simulink model "vehicle_SSC"  (R2022a)
settings: Solver=VariableStepAuto  StartTime=0.0  StopTime=10.0  RelTol=1e-3
PreLoadFcn:
  | vehicleObject = vehicle.ParallelSUV;
libraries: fl_lib x21, nesl_utility x9, sdl_lib x6
settings Model: Creator=grouleau  LastModifiedBy=grouleau

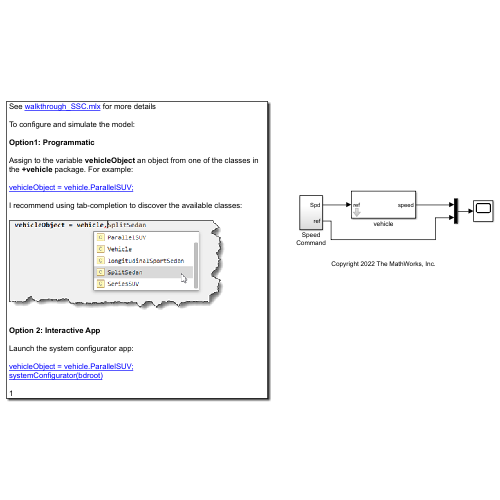
[thumbnail: Simulink's stored preview of the top-level diagram]
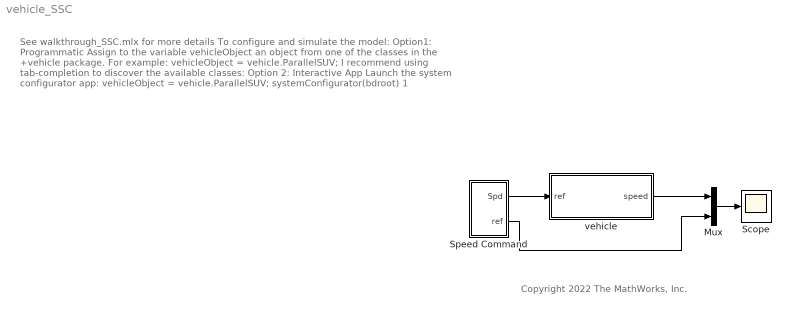
== system vehicle_SSC ==
  note: See walkthrough_SSC.mlx for more details
      |
      | To configure and simulate the model:
      |
      | Option1: Programmatic
      |
      | Assign to the variable vehicleObject an object from one of the classes in the +vehicle package. For example:
      |
      | vehicleObject = vehicle.ParallelSUV;
      |
      | I recommend using tab-completion to discover the available classes:
      |
      | Option 2: Interactive App
      |
      | Launch the system configurator app:
      |
      | vehicleObject = vehicle.ParallelSUV;
      | systemConfigurator(bdroot)
      |
      | 1
  note: Copyright 2022 The MathWorks, Inc.
  Mux : Mux  Inputs=2
  Scope : Scope
  Speed Command : Subsystem
  vehicle : Subsystem  mask(slPart){obj=vehicleObject}
      mask prompts: obj "slPart Object:"
      mask help: This subsystem implements a simplified vehicle with multiple hybrid drivetrain and parameterizations. To configure the vehicle, assign an object instantiated from one of the class in the "+vehicle" folder.
      mask init:
      | obj.maskInit(gcb);
      mask DialogControl Control2 Prompt: See walkthrough_SSC.mlx for more examples
      mask DialogControl Control2 Callback: open('walkthrough_SSC.mlx')
      mask DialogControl Container3 Prompt: Example
      mask DialogControl Control3 Prompt: vehicleObject = vehicle.ParallelSUV;
      mask DialogControl Control3 Callback: vehicleObject = vehicle.ParallelSUV;
  wires:
  Speed Command/1(Spd) -> vehicle/1(ref)
  Mux/1 -> Scope/1
  vehicle/1(speed) -> Mux/1
  Speed Command/2(ref) -> Mux/2

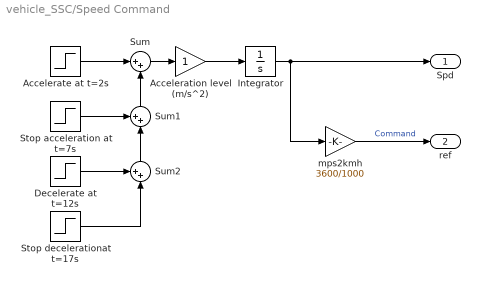
== system vehicle_SSC/Speed Command ==
  Accelerate at t=2s : Step  Time=2  SampleTime=0
  Acceleration level (m/s^2) : Gain
  Decelerate at t=12s : Step  Time=12  After=-1  SampleTime=0
  Integrator : Integrator  InitialCondition=15
  Stop acceleration at t=7s : Step  Time=7  After=-1  SampleTime=0
  Stop decelerationat t=17s : Step  Time=17  SampleTime=0
  Sum : Sum  Inputs=|++
  Sum1 : Sum  Inputs=++|
  Sum2 : Sum  Inputs=++|
  mps2kmh : Gain  Gain=3600/1000
  Spd : Outport  VectorParamsAs1DForOutWhenUnconnected=off
  ref : Outport  Port=2  VectorParamsAs1DForOutWhenUnconnected=off
  wires:
  Integrator/1 -> mps2kmh/1, Spd/1
  mps2kmh/1 -> ref/1  "Command"
  Stop decelerationat t=17s/1 -> Sum2/2
  Decelerate at t=12s/1 -> Sum2/1
  Acceleration level (m/s^2)/1 -> Integrator/1
  Sum2/1 -> Sum1/2
  Sum1/1 -> Sum/2
  Stop acceleration at t=7s/1 -> Sum1/1
  Sum/1 -> Acceleration level (m/s^2)/1
  Accelerate at t=2s/1 -> Sum/1

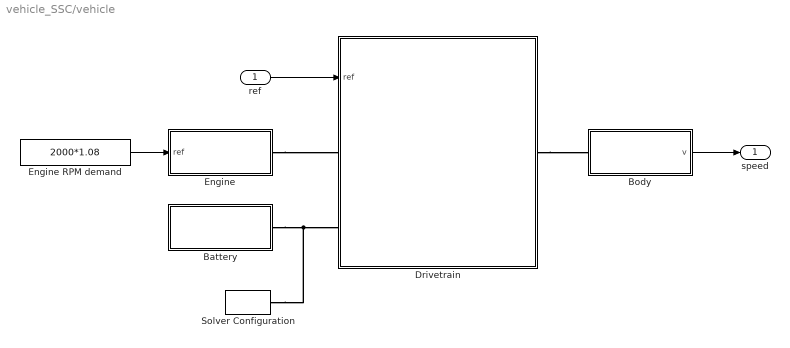
== system vehicle_SSC/vehicle ==
  ref : Inport
  Battery : Subsystem  mask(slPart){obj=obj.Battery}
      mask prompts: obj "slPart Object:"
      mask help: Container block for all slPart blocks
      mask init:
      | obj.maskInit(gcb);
  Body : Subsystem  mask(slPart){obj=obj.Body}
      mask prompts: obj "slPart Object:"
      mask help: Container block for all slPart blocks
      mask init:
      | obj.maskInit(gcb);
  Drivetrain : Subsystem  Variant=on  VariantControlMode=label  LabelModeActiveChoice=drivetrain.Parallel  mask(slPart){obj=obj.Drivetrain}
      mask prompts: obj "slPart Object:"
      mask help: Container block for all slPart blocks
      mask init:
      | obj.maskInit(gcb);
  Engine : Subsystem  mask(slPart){obj=obj.Engine}
      mask prompts: obj "slPart Object:"
      mask help: Container block for all slPart blocks
      mask init:
      | obj.maskInit(gcb);
  Engine RPM demand : Constant  Value=2000*1.08
  Solver Configuration : nesl_utility/Solver Configuration  PhysicalDomain=network_engine_domain  SubClassName=solver  LeftPortType=input  RightPortType=generic  Tones=[]  Harmonics=[]  SimulateNoise=off  Profile=off  UseLocalSampling=off  EnableSwitchedLinearOptims=on  FrequencyDomain=off  UseCCode=off  RelTol=0.001  AbsTol=1e-06  MinStep=1e-09  ToWorkspace=off  RevertToSquareIcSolve=off  NumHomotopyIterations=100  PhasorMode=off  PhasorModeNumHarmonics=1  IndexReductionMethod=DerivativeReplacement  DoDC=off  ResidualTolerance=1e-9  UseLocalSolver=off  LocalSolverChoice=NE_PARTITIONING_ADVANCER  LocalSolverSampleTime=0.005  DoFixedCost=off  MaxNonlinIter=5  MaxModeIter=2  ComputeImpulses=off  ImpulseIterations=2  LinearAlgebra=auto  LinearAlgebraNumThread=0  EquationFormulation=NE_TIME_EF  DelaysMemoryBudget=1024  AutomaticFiltering=on  FilteringTimeConstant=0.001  PartitionStorageMethod=EXHAUSTIVE  PartitionMemoryBudget=1024  PartitionMethod=ROBUST
      settings: SourceProductBaseCode=PW,SS
  speed : Outport
  wires:
  Body/1(v) -> speed/1
  ref/1 -> Drivetrain/1(ref)
  Engine RPM demand/1 -> Engine/1(ref)
  connections:
  Engine/RConn1 -- Drivetrain/LConn1
  Battery/RConn1 -- Solver Configuration/RConn1 -- Drivetrain/LConn2
  Drivetrain/RConn1 -- Body/LConn1

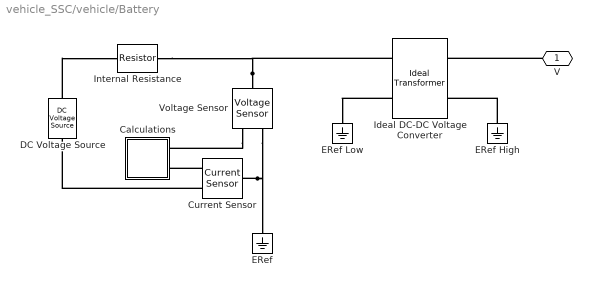
== system vehicle_SSC/vehicle/Battery ==
  Calculations : Subsystem
  Current Sensor : fl_lib/Electrical/Electrical Sensors/Current Sensor
  DC Voltage Source : fl_lib/Electrical/Electrical Sources/DC Voltage Source  v0=obj.BatteryVoltage V
  ERef : fl_lib/Electrical/Electrical Elements/Electrical Reference
  ERef High : fl_lib/Electrical/Electrical Elements/Electrical Reference
  ERef Low : fl_lib/Electrical/Electrical Elements/Electrical Reference
  Ideal DC-DC Voltage Converter : fl_lib/Electrical/Electrical Elements/Ideal Transformer  n=obj.OutputVoltage/obj.BatteryVoltage  i1_specify=off  i1_priority=None  i1=0 A  i1_nominal_specify=off  i1_nominal_unit=A  i1_nominal_value=1  v1_specify=off  v1_priority=None  v1=0 V  v1_nominal_specify=off  v1_nominal_unit=V  v1_nominal_value=1  i2_specify=off  i2_priority=None  i2=0 A  i2_nominal_specify=off  i2_nominal_unit=A  i2_nominal_value=1  v2_specify=off  v2_priority=None  v2=0 V  v2_nominal_specify=off  v2_nominal_unit=V  v2_nominal_value=1
      settings: SourceProductBaseCode=SS
  Internal Resistance : fl_lib/Electrical/Electrical Elements/Resistor  R=0.05 Ohm  i_specify=off  i_priority=High  i=0 A  i_nominal_specify=off  i_nominal_unit=A  i_nominal_value=1  v_specify=off  v_priority=High  v=0 V  v_nominal_specify=off  v_nominal_unit=V  v_nominal_value=1
  Voltage Sensor : fl_lib/Electrical/Electrical Sensors/Voltage Sensor
  V : PMIOPort  Side=Right
  connections:
  Current Sensor/LConn1 -- ERef/LConn1 -- Voltage Sensor/RConn2
  Voltage Sensor/LConn1 -- Internal Resistance/RConn1 -- Ideal DC-DC Voltage Converter/LConn1
  Current Sensor/RConn2 -- DC Voltage Source/RConn1
  Ideal DC-DC Voltage Converter/LConn2 -- ERef Low/LConn1
  Voltage Sensor/RConn1 -- Calculations/LConn1
  DC Voltage Source/LConn1 -- Internal Resistance/LConn1
  ERef High/LConn1 -- Ideal DC-DC Voltage Converter/RConn2
  Current Sensor/RConn1 -- Calculations/LConn2
  V/RConn1 -- Ideal DC-DC Voltage Converter/RConn1

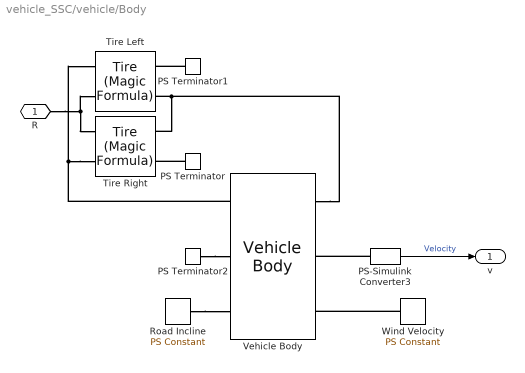
== system vehicle_SSC/vehicle/Body ==
  PS Terminator : fl_lib/Physical Signals/Sinks/PS Terminator
      settings: SourceProductBaseCode=PW,SS,VE
  PS Terminator1 : fl_lib/Physical Signals/Sinks/PS Terminator
      settings: SourceProductBaseCode=PW,SS,VE
  PS Terminator2 : fl_lib/Physical Signals/Sinks/PS Terminator
      settings: SourceProductBaseCode=PW,SS,VE
  PS-Simulink Converter3 : nesl_utility/PS-Simulink Converter  PhysicalDomain=network_engine_domain  SubClassName=ps_output  LeftPortType=input  RightPortType=output  PseudoPeriodic=off  Frequencies=[]  VectorFormat=1-D array  Unit=km/hr  AffineConversion=off
      settings: SourceProductBaseCode=PW,SS
  Road Incline : fl_lib/Physical Signals/Sources/PS Constant  constant=0
  Tire Left : sdl_lib/Tires & Vehicles/Tire (Magic Formula)  parameterization=sdl.enum.magic_tire_model.peak  F_z1=3000 N  F_x1=3500 N  kappa1=10  B_m=10  C_m=1.9  D_m=1  E_m=0.97  fz0=4e+3 N  p_Cx=1.685  p_Dx=[ 1.21 -0.037 ]  p_Ex=[ 0.344 0.095 -0.02 0 ]  p_Kx=[ 21.51 -0.163 0.245 ]  p_Hx=[ -0.002 0.002 ]  p_Vx=[ 0 0 ]  r_e=obj.WheelRadius m  model_compliance=sdl.enum.compliance.off  stiffness=1e+6 N/m  damping=1000 N/(m/s)  model_inertia=sdl.enum.model_inertia.on  inertia=1e-2 kg*m^2  initial_velocity=obj.InitialVelocity/obj.WheelRadius rad/s  model_resistance=simscape.enum.onoff.off  resistance_model=sdl.enum.rollingResistanceParameterization.constant  coeff=0.015  p_tire=2.5e+5 Pa  alpha=-0.003  beta=0.97  coeff_a=0.008399999999999999  coeff_b=6.2e-4 s/m  coeff_c=1.6e-4 s^2/m^2  v_thr=0.001 m/s  v_tr_thr=0.1 m/s
  Tire Right : sdl_lib/Tires & Vehicles/Tire (Magic Formula)  parameterization=sdl.enum.magic_tire_model.peak  F_z1=3000 N  F_x1=3500 N  kappa1=10  B_m=10  C_m=1.9  D_m=1  E_m=0.97  fz0=4e+3 N  p_Cx=1.685  p_Dx=[ 1.21 -0.037 ]  p_Ex=[ 0.344 0.095 -0.02 0 ]  p_Kx=[ 21.51 -0.163 0.245 ]  p_Hx=[ -0.002 0.002 ]  p_Vx=[ 0 0 ]  r_e=obj.WheelRadius m  model_compliance=sdl.enum.compliance.off  stiffness=1e+6 N/m  damping=1000 N/(m/s)  model_inertia=sdl.enum.model_inertia.on  inertia=1e-2 kg*m^2  initial_velocity=obj.InitialVelocity/obj.WheelRadius rad/s  model_resistance=simscape.enum.onoff.off  resistance_model=sdl.enum.rollingResistanceParameterization.constant  coeff=0.015  p_tire=2.5e+5 Pa  alpha=-0.003  beta=0.97  coeff_a=0.008399999999999999  coeff_b=6.2e-4 s/m  coeff_c=1.6e-4 s^2/m^2  v_thr=0.001 m/s  v_tr_thr=0.1 m/s
  Vehicle Body : sdl_lib/Tires & Vehicles/Vehicle Body  mass=obj.Mass kg  n_w=2  x_f=1.4 m  x_r=1.6 m  y_c=0.5 m  mass_var=simscape.enum.onoff.off  g=9.81 m/s^2  liftoff_warning=simscape.enum.onoff.off  area=3 m^2  Cd=0.4  rho=1.18 kg/m^3  model_pitch=simscape.enum.onoff.off  inertia=4000 kg*m^2  suspension_model=sdl.enum.linearTLU.linear  k_f=1e4 N/m  b_f=1e4 N/(m/s)  k_r=1e4 N/m  b_r=1e4 N/(m/s)  k_f_TLU=[-2000, -1000, 0, 1000, 2000] N  x_f_TLU=[-.4, -.2, 0, .2, .4] m  b_f_TLU=[-200, -100, 0, 100, 200] N  v_f_TLU=[-4, -2, 0, 2, 4] m/s  k_r_TLU=[-2000, -1000, 0, 1000, 2000] N  x_r_TLU=[-.4, -.2, 0, .2, .4] m  b_r_TLU=[-200, -100, 0, 100, 200] N  v_r_TLU=[-4, -2, 0, 2, 4] m/s  interp_method=simscape.enum.interpolation.linear  extrap_method=simscape.enum.extrapolation.linear  model_hardstop=simscape.enum.onoff.off  upper_bound_f=.25 m  lower_bound_f=-.25 m  stop_k_f=1e6 N/m  stop_b_f=150 N/(m/s)  upper_bound_r=.25 m  lower_bound_r=-.25 m  stop_k_r=1e6 N/m  stop_b_r=150 N/(m/s)  initial_pitch=0 rad  initial_pitch_rate=0 rad/s  v_specify=on  v_priority=High  v=obj.InitialVelocity m/s  v_nominal_specify=off  v_nominal_unit=m/s  v_nominal_value=1
  Wind Velocity : fl_lib/Physical Signals/Sources/PS Constant  constant=0
  R : PMIOPort  Side=Left
  v : Outport  VectorParamsAs1DForOutWhenUnconnected=off
  wires:
  PS-Simulink Converter3/1 -> v/1  "Velocity"
  connections:
  Vehicle Body/LConn1 -- Tire Right/RConn2 -- Tire Left/RConn2
  R/RConn1 -- Tire Left/LConn2 -- Tire Right/LConn2
  Tire Right/LConn1 -- Tire Left/LConn1 -- Vehicle Body/RConn1
  Wind Velocity/RConn1 -- Vehicle Body/LConn3
  Road Incline/RConn1 -- Vehicle Body/RConn3
  PS-Simulink Converter3/LConn1 -- Vehicle Body/LConn2
  PS Terminator/LConn1 -- Tire Right/RConn1
  PS Terminator1/LConn1 -- Tire Left/RConn1
  PS Terminator2/LConn1 -- Vehicle Body/RConn2

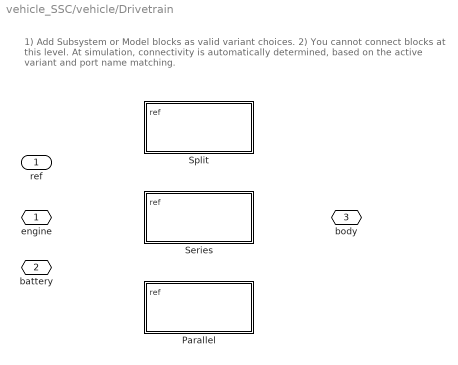
== system vehicle_SSC/vehicle/Drivetrain ==
  note: 1) Add Subsystem or Model blocks as valid variant choices.
      | 2) You cannot connect blocks at this level. At simulation, connectivity is automatically
      | determined, based on the active variant and port name matching.
  ref : Inport
  Parallel : Subsystem  VariantControl=drivetrain.Parallel
  Series : Subsystem  VariantControl=drivetrain.Series
  Split : Subsystem  VariantControl=drivetrain.Split
  engine : PMIOPort  Side=Left
  battery : PMIOPort  Port=2  Side=Left
  body : PMIOPort  Port=3  Side=Right

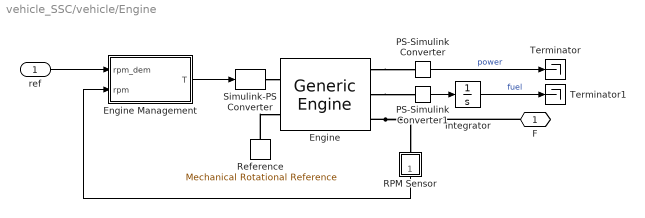
== system vehicle_SSC/vehicle/Engine ==
  ref : Inport
  Engine : sdl_lib/Engines & Motors/Generic Engine  model_parameterization=sdl.enum.engineParameterization.polynomial  engine_type=sdl.enum.engineType.SI  P_max=obj.MaximumPower kW  w_P_max=5500 rpm  w_max=7000 rpm  w_min=500 rpm  w_tab=[ 500 1000 2e+3 3e+3 4e+3 5e+3 6e+3 7e+3 ] rpm  trq_tab=[ 380 380 380 380 350 280 200 80 ] N*m  pwr_tab=[ 2e+4 4e+4 7.8e+4 1.2e+5 1.45e+5 1.48e+5 1.25e+5 6e+4 ] W  interp_method=simscape.enum.interpolation.linear  model_inertia=sdl.enum.model_inertia.on  inertia=0.2 kg*m^2  initial_velocity=obj.Initial_rpm rpm  model_time_constant=sdl.enum.lagOffOn.on  time_constant=0.2 s  T0=0.15  w_thr=20 rpm  fc_model=sdl.enum.fuel_consumption_model.BSFCSpeedBMEP  fc_per_rev=25 mg/rev  fc_w_tab=[ 1000 2e+3 3e+3 4e+3 5e+3 6e+3 ] rpm  fc_trq_tab=[ 0 80 160 200 240 320 360 400 ] N*m  fc_tab=[ 0.5 0.9 1.4 1.6 1.9 2.7 3.4 4.4; 1 1.7 2.7 3.1 3.6 5 6 7.4; 1.4 2.7 4 4.8 5.6 7.5 8.5 10.5; 2 3.6 5.8 6.7 8 10.4 11.7 13.3; 2.5 4.8 7.9 9.4 10.8 14 16.2 18.6; 3.1 6 10.3 11.9 13.8 18.4 22 26.5 ] g/s  bmep_tab=[ 0 250 500 625 750 1000 1.15e+3 1.25e+3 ] kPa  bsfc_tab=[ 410 380 300 280 270 290 320 380; 410 370 290 270 260 270 285 320; 415 380 290 275 265 270 270 300; 420 390 310 290 285 280 280 285; 430 410 340 320 310 300 310 320; 450 430 370 340 330 330 350 380 ] g/(hr*kW)  fc_interp_method=simscape.enum.interpolation.linear  idle_speed=simscape.enum.onoff.off  idle_speed_reference=1000 rpm  tau_controller=1 s  idle_w_thr=1 rpm  redline=simscape.enum.onoff.off  redline_speed=5000 rpm  tau_redline=1 s  redline_w_thr=1 rpm  displaced_volume=400 cm^3  rev_per_cycle=2
      settings: SourceProductBaseCode=LD  InternalSimscapePortConfiguration="{\"Bottom\":[],\"Left\":[{\"id\":\"T\",\"label\":\"T\",\"type\":\"input\"},{\"id\":\"B\",\"label\":\"B\",\"type\":\"foundation.mechanical.rotational.rotational\"}],\"Right\":[{\"id\":\"P\",\"label\":\"P\",\"type\":\"output\"},{\"id\":\"FC\",\"label\":\"FC\",\"type\":\"output\"},{\"id\":\"F\",\"label\":\"F\",\"type\":\"foundation.mechanical.rotational.rotational\"}],\"Top\":[]}"
  Engine Management : Subsystem
  Integrator : Integrator
  PS-Simulink Converter : nesl_utility/PS-Simulink Converter  PhysicalDomain=network_engine_domain  SubClassName=ps_output  LeftPortType=input  RightPortType=output  PseudoPeriodic=off  Frequencies=[]  VectorFormat=1-D array  Unit=inherit  AffineConversion=off
      settings: SourceProductBaseCode=PW,SS
  PS-Simulink Converter1 : nesl_utility/PS-Simulink Converter  PhysicalDomain=network_engine_domain  SubClassName=ps_output  LeftPortType=input  RightPortType=output  PseudoPeriodic=off  Frequencies=[]  VectorFormat=1-D array  Unit=inherit  AffineConversion=off
      settings: SourceProductBaseCode=PW,SS
  RPM Sensor : Subsystem
      mask Display: disp('S');
  Reference : fl_lib/Mechanical/Rotational Elements/Mechanical Rotational Reference
  Simulink-PS Converter : nesl_utility/Simulink-PS Converter  PhysicalDomain=network_engine_domain  SubClassName=ps_input  LeftPortType=input  RightPortType=output  PseudoPeriodic=off  Frequencies=[]  NoiseDistribution=none  NoiseParameters=[]  Unit=1  AffineConversion=off  FilteringAndDerivatives=zero  SimscapeFilterOrder=1  InputFilterTimeConstant=.001  UdotUserProvided=0
      settings: SourceProductBaseCode=PW,SS
  Terminator : Terminator
  Terminator1 : Terminator
  F : PMIOPort  Side=Right
  wires:
  Integrator/1 -> Terminator1/1  "fuel"
  RPM Sensor/1(rpm) -> Engine Management/2(rpm)
  Engine Management/1(T) -> Simulink-PS Converter/1
  PS-Simulink Converter/1 -> Terminator/1  "power"
  PS-Simulink Converter1/1 -> Integrator/1
  ref/1 -> Engine Management/1(rpm_dem)
  connections:
  Simulink-PS Converter/RConn1 -- Engine/LConn1
  Engine/RConn1 -- PS-Simulink Converter/LConn1
  Engine/RConn2 -- PS-Simulink Converter1/LConn1
  Reference/LConn1 -- Engine/LConn2
  Engine/RConn3 -- RPM Sensor/LConn1 -- F/RConn1

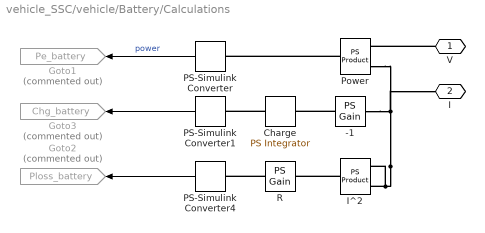
== system vehicle_SSC/vehicle/Battery/Calculations ==
  -1 : fl_lib/Physical Signals/Functions/PS Gain  gain=-1
  Charge : fl_lib/Physical Signals/Linear Operators/PS Integrator  reset_method=foundation.enum.IntegratorResetSpec.None  initial_condition_spec=foundation.enum.IntegratorICSpec.Internal  x0=150 A*hr
      settings: SourceProductBaseCode=SS
  Goto1 : Goto  Commented=on  GotoTag=Pe_battery  TagVisibility=global
  Goto2 : Goto  Commented=on  GotoTag=Ploss_battery  TagVisibility=global
  Goto3 : Goto  Commented=on  GotoTag=Chg_battery  TagVisibility=global
  I^2 : fl_lib/Physical Signals/Functions/PS Product
  PS-Simulink Converter : nesl_utility/PS-Simulink Converter  PhysicalDomain=network_engine_domain  SubClassName=ps_output  LeftPortType=input  RightPortType=output  PseudoPeriodic=off  Frequencies=[]  VectorFormat=1-D array  Unit=kW  AffineConversion=off
      settings: SourceProductBaseCode=PW,SS
  PS-Simulink Converter1 : nesl_utility/PS-Simulink Converter  PhysicalDomain=network_engine_domain  SubClassName=ps_output  LeftPortType=input  RightPortType=output  PseudoPeriodic=off  Frequencies=[]  VectorFormat=1-D array  Unit=A*hr  AffineConversion=off
      settings: SourceProductBaseCode=PW,SS
  PS-Simulink Converter4 : nesl_utility/PS-Simulink Converter  PhysicalDomain=network_engine_domain  SubClassName=ps_output  LeftPortType=input  RightPortType=output  PseudoPeriodic=off  Frequencies=[]  VectorFormat=1-D array  Unit=kW  AffineConversion=off
      settings: SourceProductBaseCode=PW,SS
  Power : fl_lib/Physical Signals/Functions/PS Product
  R : fl_lib/Physical Signals/Functions/PS Gain  gain=0.05 V/A
  V : PMIOPort  Side=Left
  I : PMIOPort  Port=2  Side=Left
  wires:
  PS-Simulink Converter4/1 -> Goto2/1
  PS-Simulink Converter1/1 -> Goto3/1
  PS-Simulink Converter/1 -> Goto1/1  "power"
  connections:
  -1/RConn1 -- Charge/LConn1
  R/RConn1 -- PS-Simulink Converter4/LConn1
  I^2/RConn1 -- R/LConn1
  I^2/LConn2 -- I/RConn1 -- Power/LConn2 -- -1/LConn1 -- I^2/LConn1
  V/RConn1 -- Power/LConn1
  Power/RConn1 -- PS-Simulink Converter/LConn1
  Charge/RConn1 -- PS-Simulink Converter1/LConn1

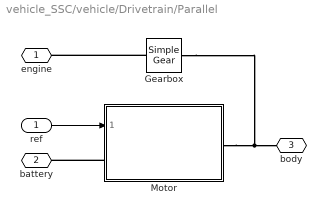
== system vehicle_SSC/vehicle/Drivetrain/Parallel ==
  ref : Inport
  Gearbox : sdl_lib/Gears/Simple Gear  ratio=4.27  rotation_direction=sdl.enum.shaftOutputDirection.same  friction_model=sdl.enum.gear_efficiencies_load.constant  T_noload=0.1 N*m  T_nom=5 N*m  efficiency_nom=0.8  efficiency=0.95  temperature_TLU=[ 280 300 320 ] K  load_TLU=[ 1 5 10 ] N*m  efficiency_TLU=[ 0.95 0.9 0.85 ]  efficiency_TLU2=[ 0.85 0.8 0.75; 0.95 0.9 0.85; 0.85 0.8 0.7 ]  w_thr=0.01 rad/s  pwr_thr=0.001 W  backlash_model=sdl.enum.backlashModel.Off  backlash_distance=1e-3 mm  x0=0 mm  r_base=0.1 m  hardstop_model=simscape.enum.hardstop.smooth  transition=1e-4 mm  backlash_stiffness=1e7 N/m  backlash_damping=1e6 N/(m/s)  e=0  v_tol=0.001 m/s  mu_visc=[ 0 0 ] N*m/(rad/s)  enable_faults=simscape.enum.onoff.off  efficiency_fault=0.05  external_fault=simscape.enum.onoff.off  temporal_fault=simscape.enum.onoff.off  fault_time=5 s  fault_angles=pi / 12 rad  report_fault=simscape.enum.assert.action.none  thermal_mass=50 J/K  temperature_specify=off  temperature_priority=High  temperature=300 K  temperature_nominal_specify=off  temperature_nominal_unit=K  temperature_nominal_value=1  x_backlash_specify=off  x_backlash_priority=None  x_backlash=0 mm  x_backlash_nominal_specify=off  x_backlash_nominal_unit=mm  x_backlash_nominal_value=1  f_hardstop_specify=off  f_hardstop_priority=None  f_hardstop=0 N  f_hardstop_nominal_specify=off  f_hardstop_nominal_unit=N  f_hardstop_nominal_value=1  v_backlash_specify=off  v_backlash_priority=None  v_backlash=0 m/s  v_backlash_nominal_specify=off  v_backlash_nominal_unit=m/s  v_backlash_nominal_value=1
  Motor : Subsystem  ReferencedSubsystem=motor_ss  obj=obj.Motor
  engine : PMIOPort  Side=Left
  battery : PMIOPort  Port=2  Side=Left
  body : PMIOPort  Port=3  Side=Right
  wires:
  ref/1 -> Motor/1
  connections:
  Motor/RConn1 -- Gearbox/RConn1 -- body/RConn1
  Motor/LConn1 -- battery/RConn1
  Gearbox/LConn1 -- engine/RConn1

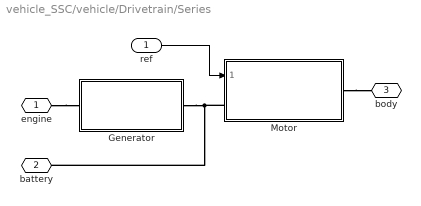
== system vehicle_SSC/vehicle/Drivetrain/Series ==
  ref : Inport
  Generator : Subsystem  ReferencedSubsystem=generator_ss  obj=obj.Generator
  Motor : Subsystem  ReferencedSubsystem=motor_ss  obj=obj.Motor
  engine : PMIOPort  Side=Left
  battery : PMIOPort  Port=2  Side=Left
  body : PMIOPort  Port=3  Side=Right
  wires:
  ref/1 -> Motor/1
  connections:
  engine/RConn1 -- Generator/LConn1
  Generator/RConn1 -- Motor/LConn1 -- battery/RConn1
  Motor/RConn1 -- body/RConn1

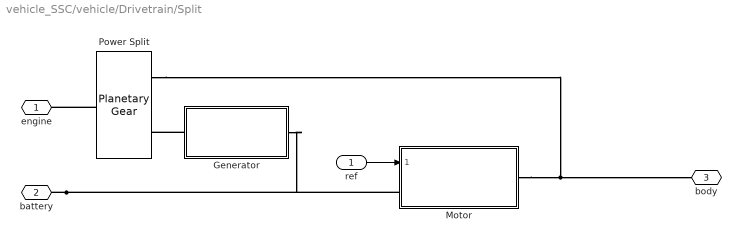
== system vehicle_SSC/vehicle/Drivetrain/Split ==
  ref : Inport
  Generator : Subsystem  ReferencedSubsystem=generator_ss  obj=obj.Generator
  Motor : Subsystem  ReferencedSubsystem=motor_ss  obj=obj.Motor
  Power Split : sdl_lib/Gears/Planetary Gear  rs_ratio=2  friction_model=2  efficiency=[ 0.96 0.98 ]  temperature_TLU=[ 280 300 320 ] K  efficiency_sp_TLU=[ 0.95 0.9 0.85 ]  efficiency_rp_TLU=[ 0.95 0.9 0.85 ]  pwr_thr=[ 0.001 0.001 ] W  mu_visc=[ 0 0 ] N*m/(rad/s)  model_inertia=0  planet_inertia=0.001 kg*m^2  thermal_mass=50 J/K  T_init=300 K
      settings: SourceProductBaseCode=LD
  engine : PMIOPort  Side=Left
  battery : PMIOPort  Port=2  Side=Left
  body : PMIOPort  Port=3  Side=Right
  wires:
  ref/1 -> Motor/1
  connections:
  Power Split/RConn1 -- body/RConn1 -- Motor/RConn1
  battery/RConn1 -- Motor/LConn1 -- Generator/RConn1
  Generator/LConn1 -- Power Split/RConn2
  Power Split/LConn1 -- engine/RConn1

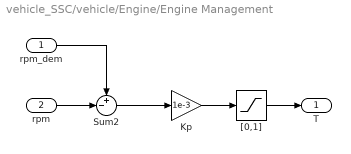
== system vehicle_SSC/vehicle/Engine/Engine Management ==
  rpm_dem : Inport
  rpm : Inport  Port=2
  Kp : Gain  Gain=1e-3  SaturateOnIntegerOverflow=on  OutDataTypeStr=Inherit: Same as input  ParamDataTypeStr=Inherit: Same as input
  Sum2 : Sum  Inputs=+-|  InputSameDT=on  SaturateOnIntegerOverflow=on  OutDataTypeStr=Inherit: Same as first input
  "[0,1]" : Saturate  UpperLimit=1  LowerLimit=0
  T : Outport  VectorParamsAs1DForOutWhenUnconnected=off
  wires:
  rpm/1 -> Sum2/2
  rpm_dem/1 -> Sum2/1
  Sum2/1 -> Kp/1
  Kp/1 -> "[0,1]"/1
  "[0,1]"/1 -> T/1

== system vehicle_SSC/vehicle/Engine/RPM Sensor ==
  Ideal Rotational Motion Sensor : fl_lib/Mechanical/Mechanical Sensors/Ideal Rotational Motion Sensor  wrap_angle=simscape.enum.onoff.off  offset=0 rad
  MRR : fl_lib/Mechanical/Rotational Elements/Mechanical Rotational Reference
  PS2S : nesl_utility/PS-Simulink Converter  PhysicalDomain=network_engine_domain  SubClassName=ps_output  LeftPortType=input  RightPortType=output  PseudoPeriodic=off  Frequencies=[]  VectorFormat=1-D array  Unit=rpm  AffineConversion=off
      settings: SourceProductBaseCode=PW,SS
  Sensor dynamics : TransferFcn  Denominator=[0.01 1]
  F : PMIOPort  Side=Left
  rpm : Outport  VectorParamsAs1DForOutWhenUnconnected=off
  wires:
  PS2S/1 -> Sensor dynamics/1
  Sensor dynamics/1 -> rpm/1
  connections:
  F/RConn1 -- Ideal Rotational Motion Sensor/LConn1
  Ideal Rotational Motion Sensor/RConn2 -- PS2S/LConn1
  MRR/LConn1 -- Ideal Rotational Motion Sensor/RConn1
